simulink model "matlab2simutrial"  (R2018b)
settings: Solver=VariableStepAuto  StartTime=0.0  StopTime=10.0  RelTol=1e-3
values from neighbouring files (symbols this model uses):
  b = 12    [matlab2simutrial1.m]
  f = 8    [matlab2simutrial1.m]
  k = 16    [matlab2simutrial1.m]
  m = 2    [matlab2simutrial1.m]
settings Model: Creator=student  LastModifiedBy=student

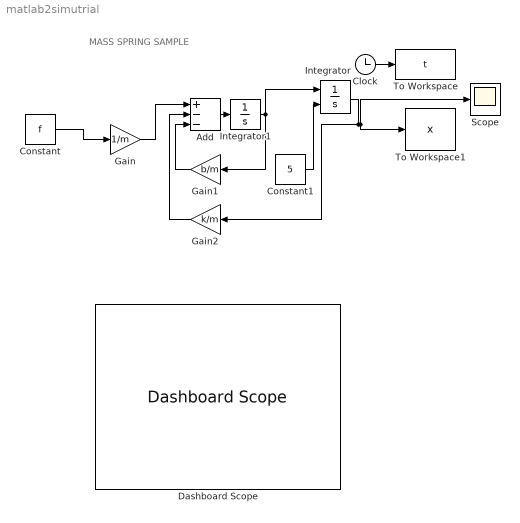
== system matlab2simutrial ==
  note: MASS SPRING SAMPLE
  Add : Sum  Inputs=+--
  Clock : Clock
  Constant : Constant  Value=f
  Constant1 : Constant  Value=5
  Dashboard Scope : DashboardScope  WebBlockId=10
  Gain : Gain  Gain=1/m
  Gain1 : Gain  Gain=b/m
  Gain2 : Gain  Gain=k/m
  Integrator : Integrator  InitialConditionSource=external
  Integrator1 : Integrator
  Scope : Scope
  To Workspace : ToWorkspace  VariableName=t  SampleTime=-1
  To Workspace1 : ToWorkspace  VariableName=x  SampleTime=-1
      settings: Save2DSignal=2-D array (concatenate along first dimension)
  wires:
  Integrator1/1 -> Gain1/1, Integrator/1
  Integrator/1 -> Gain2/1, To Workspace1/1, Scope/1
  Gain1/1 -> Add/3
  Gain2/1 -> Add/2
  Gain/1 -> Add/1
  Add/1 -> Integrator1/1
  Constant/1 -> Gain/1
  Clock/1 -> To Workspace/1
  Constant1/1 -> Integrator/2
